simulink model "test_quadruped_troting"  (Simulink 9.2)
settings: Solver=VariableStepDiscrete  StartTime=0.0  StopTime=12  FixedStep=0.001  MaxStep=0.001  RelTol=1e-10  EnableMultiTasking=on
values from neighbouring files (symbols this model uses):
  Output_file_n = r_temp___(2)    [quadruped.m]
  Plant_inputs_num = r_temp___(1)    [quadruped.m]
  Plant_outputs_num = r_temp___(1)    [quadruped.m]
  RecurDyn_model_n = r_temp___(2)    [quadruped.m]
undefined symbols (not defined in the file): Matlab_version, Output_File, RecurDyn, RecurDyn_controltimestep, RecurDyn_model
(part 1 of 2)
settings Model: Creator=admin  LastModifiedBy=ahl19
settings OptimizationCC: ExpressionDepthLimit=2147483647
settings DebuggingCC: SolverPrmCheckMsg=warning
settings GRTTargetCC: CombineOutputUpdateFcns=on  GRTInterface=off

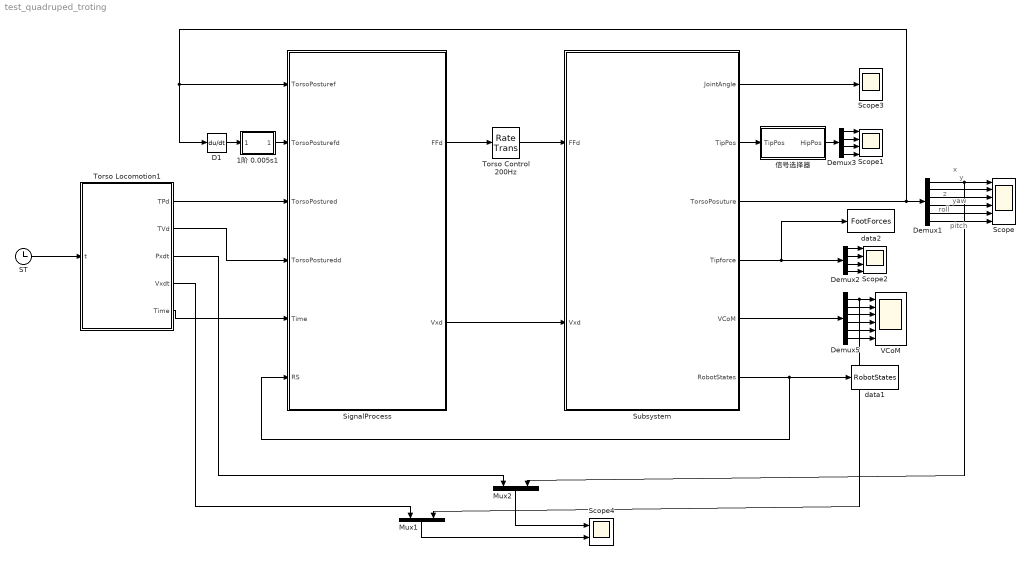
== system test_quadruped_troting ==
  note: x
  note: y
  note: z
  note: yaw
  note: roll
  note: pitch
  1阶 0.005s1 : Subsystem
  D1 : Derivative  CoefficientInTFapproximation=0.01
  Demux1 : Demux  Outputs=6
  Demux2 : Demux
  Demux3 : Demux
  Demux5 : Demux  Outputs=6
  Mux1 : Mux  Inputs=2
  Mux2 : Mux  Inputs=2
  ST : Clock
  Scope : Scope  NumInputPorts=6
  Scope1 : Scope  NumInputPorts=4
  Scope2 : Scope  NumInputPorts=4
  Scope3 : Scope
  Scope4 : Scope  NumInputPorts=2
  SignalProcess : MATLAB Function  TreatAsAtomicUnit=on
  Subsystem : Subsystem
  Torso Control 200Hz : RateTransition  OutPortSampleTime=0.005
  Torso Locomotion1 : MATLAB Function  TreatAsAtomicUnit=on
  VCoM : Scope  NumInputPorts=6
  data1 : ToWorkspace  VariableName=RobotStates  SaveFormat=Timeseries  SampleTime=-1
  data2 : ToWorkspace  VariableName=FootForces  SaveFormat=Timeseries  SampleTime=-1
  信号选择器 : MATLAB Function  TreatAsAtomicUnit=on
  wires:
  Subsystem/3(TorsoPosuture) -> Demux1/1, SignalProcess/1(TorsoPosturef), D1/1
  SignalProcess/1(FFd) -> Torso Control 200Hz/1
  Demux2/1 -> Scope2/1
  Demux2/2 -> Scope2/2
  Demux2/3 -> Scope2/3
  Demux2/4 -> Scope2/4
  Subsystem/4(Tipforce) -> Demux2/1, data2/1
  Subsystem/2(TipPos) -> 信号选择器/1(TipPos)
  Demux3/1 -> Scope1/1
  Demux3/2 -> Scope1/2
  Demux3/3 -> Scope1/3
  Demux3/4 -> Scope1/4
  Subsystem/1(JointAngle) -> Scope3/1
  信号选择器/1(HipPos) -> Demux3/1
  Torso Control 200Hz/1 -> Subsystem/1(FFd)
  Subsystem/6(RobotStates) -> data1/1, SignalProcess/6(RS)
  Subsystem/5(VCoM) -> Demux5/1
  Demux5/1 -> VCoM/1, Mux1/2
  Demux5/2 -> VCoM/2
  Demux5/3 -> VCoM/3
  Demux5/4 -> VCoM/4
  Demux5/5 -> VCoM/5
  Demux5/6 -> VCoM/6
  D1/1 -> 1阶 0.005s1/1(VT0)
  1阶 0.005s1/1(VT1) -> SignalProcess/2(TorsoPosturefd)
  SignalProcess/2(Vxd) -> Subsystem/2(Vxd)
  Demux1/1 -> Scope/1, Mux2/2
  Demux1/2 -> Scope/2
  Demux1/3 -> Scope/3
  Demux1/4 -> Scope/4
  Demux1/5 -> Scope/5
  Demux1/6 -> Scope/6
  Torso Locomotion1/5(Time) -> SignalProcess/5(Time)
  Torso Locomotion1/1(TPd) -> SignalProcess/3(TorsoPostured)
  Torso Locomotion1/2(TVd) -> SignalProcess/4(TorsoPosturedd)
  ST/1 -> Torso Locomotion1/1(t)
  Torso Locomotion1/3(Pxdt) -> Mux2/1
  Mux2/1 -> Scope4/1
  Torso Locomotion1/4(Vxdt) -> Mux1/1
  Mux1/1 -> Scope4/2

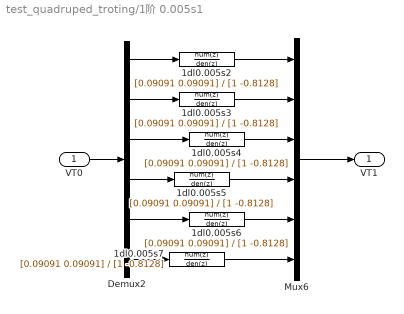
== system test_quadruped_troting/1阶 0.005s1 ==
  VT0 : Inport
  1dl0.005s{2..7} (6 alike) : DiscreteTransferFcn  Numerator=[0.09091 0.09091]  Denominator=[1 -0.8128]  SampleTime=0.001
  Demux2 : Demux  Outputs=6
  Mux6 : Mux  Inputs=6
  VT1 : Outport
  wires:
  Demux2/1 -> 1dl0.005s2/1
  Demux2/2 -> 1dl0.005s3/1
  Demux2/3 -> 1dl0.005s4/1
  Demux2/4 -> 1dl0.005s5/1
  Demux2/5 -> 1dl0.005s6/1
  Demux2/6 -> 1dl0.005s7/1
  1dl0.005s2/1 -> Mux6/1
  1dl0.005s4/1 -> Mux6/3
  1dl0.005s5/1 -> Mux6/4
  1dl0.005s6/1 -> Mux6/5
  1dl0.005s7/1 -> Mux6/6
  1dl0.005s3/1 -> Mux6/2
  Mux6/1 -> VT1/1
  VT0/1 -> Demux2/1

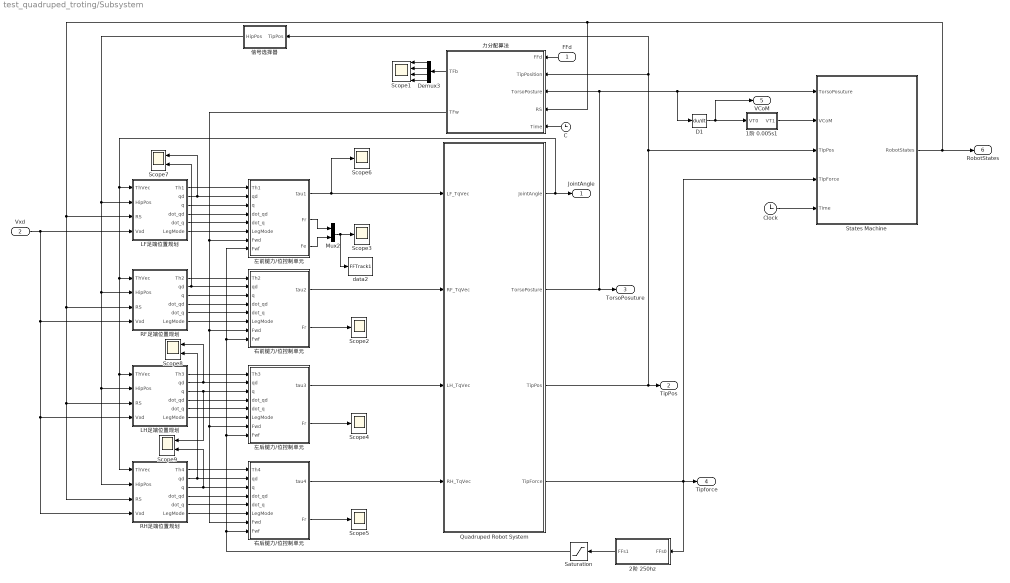
== system test_quadruped_troting/Subsystem ==
  FFd : Inport
  Vxd : Inport  Port=2
  1阶 0.005s1 : Subsystem
  2阶 250hz : Subsystem
  C : Clock
  Clock : Clock
  D1 : Derivative  CoefficientInTFapproximation=0.01
  Demux3 : Demux
  LF足端位置规划 : Subsystem
  LH足端位置规划 : Subsystem
  Mux2 : Mux  Inputs=2
  Quadruped Robot System : Subsystem
  RF足端位置规划 : Subsystem
  RH足端位置规划 : Subsystem
  Saturation : Saturate  UpperLimit=1500  LowerLimit=-1500
  Scope1 : Scope  NumInputPorts=4
  Scope{2..6} (5 alike) : Scope
  Scope7 : Scope  NumInputPorts=2
  Scope8 : Scope  NumInputPorts=2
  Scope9 : Scope  NumInputPorts=2
  States Machine : MATLAB Function  TreatAsAtomicUnit=on
  data2 : ToWorkspace  VariableName=FFTrack1  SaveFormat=Timeseries  SampleTime=-1
  信号选择器 : MATLAB Function  TreatAsAtomicUnit=on
  力分配算法 : MATLAB Function  TreatAsAtomicUnit=on
  右前腿力/位控制单元 : MATLAB Function  TreatAsAtomicUnit=on
  右后腿力/位控制单元 : MATLAB Function  TreatAsAtomicUnit=on
  左前腿力/位控制单元 : MATLAB Function  TreatAsAtomicUnit=on
  左后腿力/位控制单元 : MATLAB Function  TreatAsAtomicUnit=on
  JointAngle : Outport
  TipPos : Outport  Port=2
  TorsoPosuture : Outport  Port=3
  Tipforce : Outport  Port=4
  VCoM : Outport  Port=5
  RobotStates : Outport  Port=6
  wires:
  Quadruped Robot System/1(JointAngle) -> JointAngle/1, LF足端位置规划/1(ThVec), RF足端位置规划/1(ThVec), LH足端位置规划/1(ThVec), RH足端位置规划/1(ThVec)
  Quadruped Robot System/3(TipPos) -> TipPos/1, 信号选择器/1(TipPos), 力分配算法/2(TipPosition), States Machine/3(TipPos)
  Quadruped Robot System/2(TorsoPosture) -> TorsoPosuture/1, 力分配算法/3(TorsoPosture), States Machine/1(TorsoPosuture), D1/1
  Quadruped Robot System/4(TipForce) -> Tipforce/1, States Machine/4(TipForce), 2阶 250hz/1(FFs0)
  FFd/1 -> 力分配算法/1(FFd)
  C/1 -> 力分配算法/5(Time)
  左前腿力/位控制单元/1(tau1) -> Scope6/1, Quadruped Robot System/1(LF_TqVec)
  Demux3/1 -> Scope1/1
  Demux3/2 -> Scope1/2
  Demux3/3 -> Scope1/3
  Demux3/4 -> Scope1/4
  力分配算法/1(TFb) -> Demux3/1
  右前腿力/位控制单元/2(Fr) -> Scope2/1
  左后腿力/位控制单元/2(Fr) -> Scope4/1
  右后腿力/位控制单元/2(Fr) -> Scope5/1
  Mux2/1 -> Scope3/1, data2/1
  左前腿力/位控制单元/2(Fr) -> Mux2/1
  左前腿力/位控制单元/3(Fe) -> Mux2/2
  Clock/1 -> States Machine/5(Time)
  States Machine/1(RobotStates) -> RobotStates/1, LF足端位置规划/3(RS), LH足端位置规划/3(RS), RH足端位置规划/3(RS), RF足端位置规划/3(RS), 力分配算法/4(RS)
  LF足端位置规划/1(Th1) -> 左前腿力/位控制单元/1(Th1)
  LF足端位置规划/2(qd) -> Scope7/1, 左前腿力/位控制单元/2(qd)
  LF足端位置规划/3(q) -> 左前腿力/位控制单元/3(q)
  LF足端位置规划/4(dot_qd) -> 左前腿力/位控制单元/4(dot_qd)
  LF足端位置规划/5(dot_q) -> 左前腿力/位控制单元/5(dot_q)
  LF足端位置规划/6(LegMode) -> 左前腿力/位控制单元/6(LegMode)
  RF足端位置规划/1(Th2) -> 右前腿力/位控制单元/1(Th2)
  RF足端位置规划/2(qd) -> 右前腿力/位控制单元/2(qd), Scope7/2
  RF足端位置规划/3(q) -> 右前腿力/位控制单元/3(q)
  RF足端位置规划/4(dot_qd) -> 右前腿力/位控制单元/4(dot_qd)
  RF足端位置规划/5(dot_q) -> 右前腿力/位控制单元/5(dot_q)
  RF足端位置规划/6(LegMode) -> 右前腿力/位控制单元/6(LegMode)
  LH足端位置规划/1(Th3) -> 左后腿力/位控制单元/1(Th3)
  LH足端位置规划/2(qd) -> 左后腿力/位控制单元/2(qd), Scope8/1
  LH足端位置规划/3(q) -> 左后腿力/位控制单元/3(q), Scope9/1
  LH足端位置规划/4(dot_qd) -> 左后腿力/位控制单元/4(dot_qd)
  LH足端位置规划/5(dot_q) -> 左后腿力/位控制单元/5(dot_q)
  LH足端位置规划/6(LegMode) -> 左后腿力/位控制单元/6(LegMode)
  RH足端位置规划/1(Th4) -> 右后腿力/位控制单元/1(Th4)
  RH足端位置规划/2(qd) -> 右后腿力/位控制单元/2(qd), Scope8/2
  RH足端位置规划/3(q) -> 右后腿力/位控制单元/3(q), Scope9/2
  RH足端位置规划/4(dot_qd) -> 右后腿力/位控制单元/4(dot_qd)
  RH足端位置规划/5(dot_q) -> 右后腿力/位控制单元/5(dot_q)
  RH足端位置规划/6(LegMode) -> 右后腿力/位控制单元/6(LegMode)
  信号选择器/1(HipPos) -> LF足端位置规划/2(HipPos), RF足端位置规划/2(HipPos), LH足端位置规划/2(HipPos), RH足端位置规划/2(HipPos)
  力分配算法/2(TFw) -> 左前腿力/位控制单元/7(Fwd), 右前腿力/位控制单元/7(Fwd), 左后腿力/位控制单元/7(Fwd), 右后腿力/位控制单元/7(Fwd)
  Saturation/1 -> 右后腿力/位控制单元/8(Fwf), 左后腿力/位控制单元/8(Fwf), 右前腿力/位控制单元/8(Fwf), 左前腿力/位控制单元/8(Fwf)
  D1/1 -> 1阶 0.005s1/1(VT0), VCoM/1
  2阶 250hz/1(FFs1) -> Saturation/1
  1阶 0.005s1/1(VT1) -> States Machine/2(VCoM)
  Vxd/1 -> LF足端位置规划/4(Vxd), RF足端位置规划/4(Vxd), LH足端位置规划/4(Vxd), RH足端位置规划/4(Vxd)
  右前腿力/位控制单元/1(tau2) -> Quadruped Robot System/2(RF_TqVec)
  左后腿力/位控制单元/1(tau3) -> Quadruped Robot System/3(LH_TqVec)
  右后腿力/位控制单元/1(tau4) -> Quadruped Robot System/4(RH_TqVec)

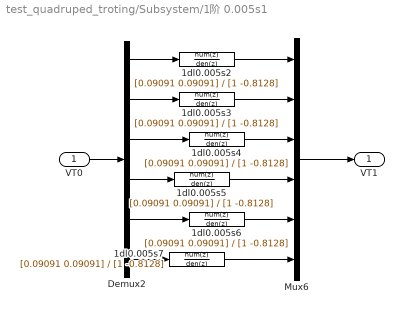
== system test_quadruped_troting/Subsystem/1阶 0.005s1 ==
  VT0 : Inport
  1dl0.005s{2..7} (6 alike) : DiscreteTransferFcn  Numerator=[0.09091 0.09091]  Denominator=[1 -0.8128]  SampleTime=0.001
  Demux2 : Demux  Outputs=6
  Mux6 : Mux  Inputs=6
  VT1 : Outport
  wires:
  Demux2/1 -> 1dl0.005s2/1
  Demux2/2 -> 1dl0.005s3/1
  Demux2/3 -> 1dl0.005s4/1
  Demux2/4 -> 1dl0.005s5/1
  Demux2/5 -> 1dl0.005s6/1
  Demux2/6 -> 1dl0.005s7/1
  1dl0.005s2/1 -> Mux6/1
  1dl0.005s4/1 -> Mux6/3
  1dl0.005s5/1 -> Mux6/4
  1dl0.005s6/1 -> Mux6/5
  1dl0.005s7/1 -> Mux6/6
  1dl0.005s3/1 -> Mux6/2
  Mux6/1 -> VT1/1
  VT0/1 -> Demux2/1

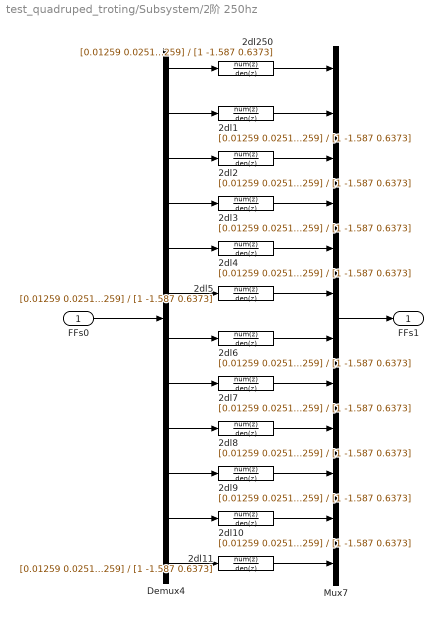
== system test_quadruped_troting/Subsystem/2阶 250hz ==
  FFs0 : Inport
  2dl{1..11,250} (12 alike) : DiscreteTransferFcn  Numerator=[0.01259 0.02519 0.01259]  Denominator=[1 -1.587 0.6373]  SampleTime=0.001
  Demux4 : Demux  Outputs=12
  Mux7 : Mux  Inputs=12
  FFs1 : Outport
  wires:
  FFs0/1 -> Demux4/1
  Mux7/1 -> FFs1/1
  Demux4/1 -> 2dl250/1
  Demux4/2 -> 2dl1/1
  Demux4/3 -> 2dl2/1
  Demux4/4 -> 2dl3/1
  Demux4/5 -> 2dl4/1
  Demux4/6 -> 2dl5/1
  Demux4/7 -> 2dl6/1
  Demux4/8 -> 2dl7/1
  Demux4/9 -> 2dl8/1
  Demux4/10 -> 2dl9/1
  Demux4/11 -> 2dl10/1
  Demux4/12 -> 2dl11/1
  2dl250/1 -> Mux7/1
  2dl1/1 -> Mux7/2
  2dl2/1 -> Mux7/3
  2dl3/1 -> Mux7/4
  2dl4/1 -> Mux7/5
  2dl5/1 -> Mux7/6
  2dl6/1 -> Mux7/7
  2dl7/1 -> Mux7/8
  2dl8/1 -> Mux7/9
  2dl9/1 -> Mux7/10
  2dl10/1 -> Mux7/11
  2dl11/1 -> Mux7/12

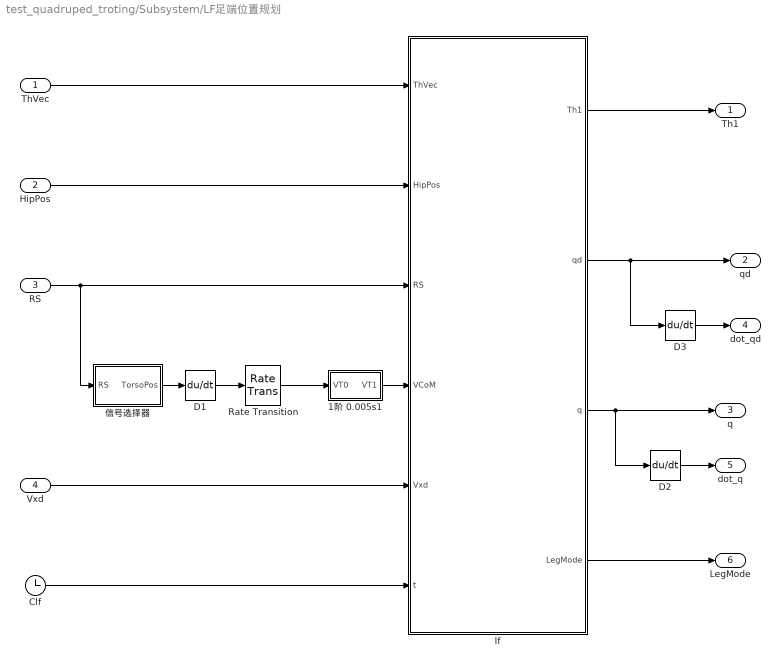
== system test_quadruped_troting/Subsystem/LF足端位置规划 ==
  ThVec : Inport
  HipPos : Inport  Port=2
  RS : Inport  Port=3
  Vxd : Inport  Port=4
  1阶 0.005s1 : Subsystem
  Clf : Clock
  D1 : Derivative  CoefficientInTFapproximation=0.01
  D2 : Derivative  CoefficientInTFapproximation=0.01
  D3 : Derivative  CoefficientInTFapproximation=0.01
  Rate Transition : RateTransition  OutPortSampleTime=0.002
  lf : MATLAB Function  TreatAsAtomicUnit=on
  信号选择器 : MATLAB Function  TreatAsAtomicUnit=on
  Th1 : Outport
  qd : Outport  Port=2
  q : Outport  Port=3
  dot_qd : Outport  Port=4
  dot_q : Outport  Port=5
  LegMode : Outport  Port=6
  wires:
  HipPos/1 -> lf/2(HipPos)
  ThVec/1 -> lf/1(ThVec)
  lf/1(Th1) -> Th1/1
  D2/1 -> dot_q/1
  D3/1 -> dot_qd/1
  Clf/1 -> lf/6(t)
  D1/1 -> Rate Transition/1
  lf/4(LegMode) -> LegMode/1
  RS/1 -> lf/3(RS), 信号选择器/1(RS)
  信号选择器/1(TorsoPos) -> D1/1
  lf/3(q) -> q/1, D2/1
  lf/2(qd) -> qd/1, D3/1
  Rate Transition/1 -> 1阶 0.005s1/1(VT0)
  1阶 0.005s1/1(VT1) -> lf/4(VCoM)
  Vxd/1 -> lf/5(Vxd)

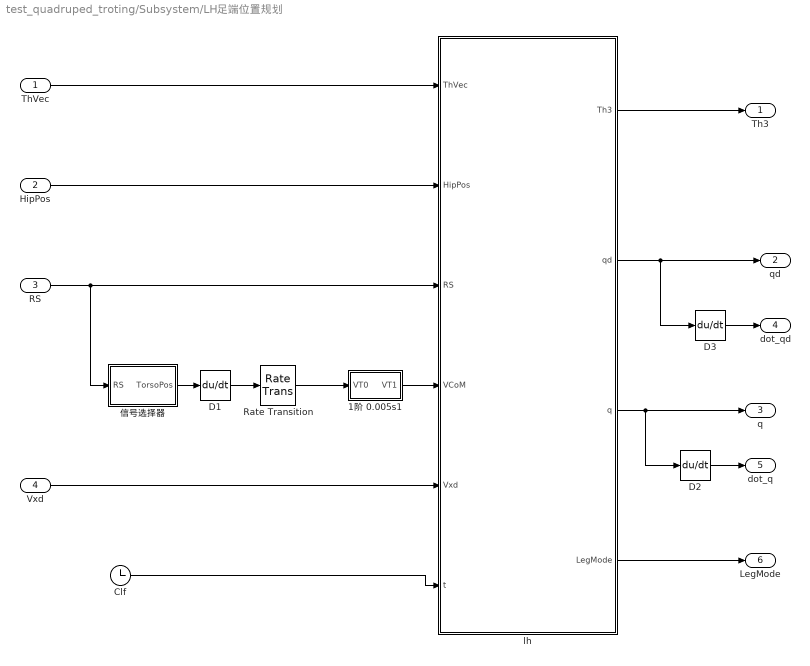
== system test_quadruped_troting/Subsystem/LH足端位置规划 ==
  ThVec : Inport
  HipPos : Inport  Port=2
  RS : Inport  Port=3
  Vxd : Inport  Port=4
  1阶 0.005s1 : Subsystem
  Clf : Clock
  D1 : Derivative  CoefficientInTFapproximation=0.01
  D2 : Derivative  CoefficientInTFapproximation=0.01
  D3 : Derivative  CoefficientInTFapproximation=0.01
  Rate Transition : RateTransition  OutPortSampleTime=0.002
  lh : MATLAB Function  TreatAsAtomicUnit=on
  信号选择器 : MATLAB Function  TreatAsAtomicUnit=on
  Th3 : Outport
  qd : Outport  Port=2
  q : Outport  Port=3
  dot_qd : Outport  Port=4
  dot_q : Outport  Port=5
  LegMode : Outport  Port=6
  wires:
  HipPos/1 -> lh/2(HipPos)
  ThVec/1 -> lh/1(ThVec)
  lh/1(Th3) -> Th3/1
  D2/1 -> dot_q/1
  D3/1 -> dot_qd/1
  Clf/1 -> lh/6(t)
  D1/1 -> Rate Transition/1
  lh/4(LegMode) -> LegMode/1
  RS/1 -> lh/3(RS), 信号选择器/1(RS)
  信号选择器/1(TorsoPos) -> D1/1
  lh/3(q) -> q/1, D2/1
  lh/2(qd) -> qd/1, D3/1
  Rate Transition/1 -> 1阶 0.005s1/1(VT0)
  1阶 0.005s1/1(VT1) -> lh/4(VCoM)
  Vxd/1 -> lh/5(Vxd)

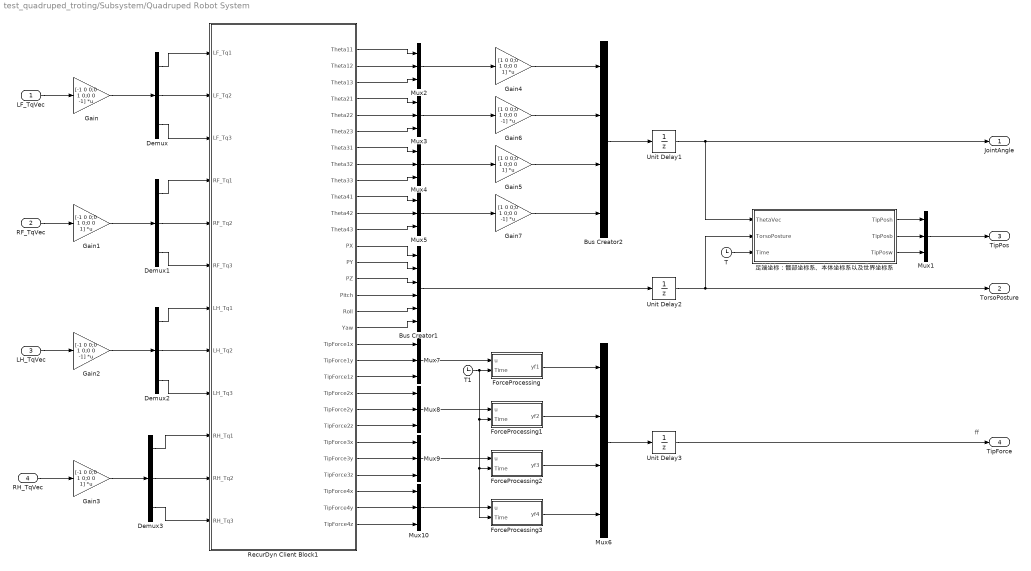
== system test_quadruped_troting/Subsystem/Quadruped Robot System ==
  note: ff
  LF_TqVec : Inport
  RF_TqVec : Inport  Port=2
  LH_TqVec : Inport  Port=3
  RH_TqVec : Inport  Port=4
  Bus Creator1 : BusCreator  Inputs=6
  Bus Creator2 : BusCreator  Inputs=4
  Demux{,1..3} (4 alike) : Demux  Outputs=3
  ForceProcessing : MATLAB Function  TreatAsAtomicUnit=on
  ForceProcessing1 : MATLAB Function  TreatAsAtomicUnit=on
  ForceProcessing2 : MATLAB Function  TreatAsAtomicUnit=on
  ForceProcessing3 : MATLAB Function  TreatAsAtomicUnit=on
  Gain : Gain  Gain=[-1 0 0;0 1 0;0 0 -1]  Multiplication=Matrix(K*u) (u vector)
  Gain1 : Gain  Gain=[-1 0 0;0 1 0;0 0 1]  Multiplication=Matrix(K*u) (u vector)
  Gain2 : Gain  Gain=[-1 0 0;0 1 0;0 0 -1]  Multiplication=Matrix(K*u) (u vector)
  Gain3 : Gain  Gain=[-1 0 0;0 1 0;0 0 1]  Multiplication=Matrix(K*u) (u vector)
  Gain4 : Gain  Gain=[1 0 0;0 1 0;0 0 1]  Multiplication=Matrix(K*u) (u vector)
  Gain5 : Gain  Gain=[1 0 0;0 1 0;0 0 1]  Multiplication=Matrix(K*u) (u vector)
  Gain6 : Gain  Gain=[1 0 0;0 1 0;0 0 -1]  Multiplication=Matrix(K*u) (u vector)
  Gain7 : Gain  Gain=[1 0 0;0 1 0;0 0 -1]  Multiplication=Matrix(K*u) (u vector)
  Mux{1..5,7..10} (9 alike) : Mux  Inputs=3
  Mux6 : Mux
  RecurDyn Client Block1 : Subsystem
      mask Display: image(imread('RecurDyn_IF3x_Client.jpg'))
  T : Clock
  T1 : Clock
  Unit Delay1 : UnitDelay  InitialCondition=[pi/2;pi/4;0;pi/2;pi/4;0;pi/2;pi/4;0;pi/2;pi/4;0]  SampleTime=0.001
  Unit Delay2 : UnitDelay  InitialCondition=[0;0.70;0;0;0;0]  SampleTime=0.001
  Unit Delay3 : UnitDelay  InitialCondition=[0;0;0;0;0;0;0;0;0;0;0;0]  SampleTime=0.001
  足端坐标：髋部坐标系、本体坐标系以及世界坐标系 : MATLAB Function  TreatAsAtomicUnit=on
  JointAngle : Outport
  TorsoPosture : Outport  Port=2
  TipPos : Outport  Port=3
  TipForce : Outport  Port=4
  wires:
  Bus Creator2/1 -> Unit Delay1/1
  Mux1/1 -> TipPos/1
  足端坐标：髋部坐标系、本体坐标系以及世界坐标系/1(TipPosh) -> Mux1/1
  足端坐标：髋部坐标系、本体坐标系以及世界坐标系/2(TipPosb) -> Mux1/2
  足端坐标：髋部坐标系、本体坐标系以及世界坐标系/3(TipPosw) -> Mux1/3
  Unit Delay1/1 -> JointAngle/1, 足端坐标：髋部坐标系、本体坐标系以及世界坐标系/1(ThetaVec)
  Unit Delay3/1 -> TipForce/1
  Unit Delay2/1 -> TorsoPosture/1, 足端坐标：髋部坐标系、本体坐标系以及世界坐标系/2(TorsoPosture)
  Mux7/1 -> ForceProcessing/1(u)
  Mux8/1 -> ForceProcessing1/1(u)
  Mux9/1 -> ForceProcessing2/1(u)
  Mux10/1 -> ForceProcessing3/1(u)
  Gain/1 -> Demux/1
  LF_TqVec/1 -> Gain/1
  RF_TqVec/1 -> Gain1/1
  LH_TqVec/1 -> Gain2/1
  RH_TqVec/1 -> Gain3/1
  Mux2/1 -> Gain4/1
  Bus Creator1/1 -> Unit Delay2/1
  Demux/2 -> RecurDyn Client Block1/2(LF_Tq2)
  RecurDyn Client Block1/1("Theta11   ") -> Mux2/1
  RecurDyn Client Block1/2("Theta12   ") -> Mux2/2
  RecurDyn Client Block1/3("Theta13   ") -> Mux2/3
  RecurDyn Client Block1/4("Theta21   ") -> Mux3/1
  RecurDyn Client Block1/5("Theta22   ") -> Mux3/2
  RecurDyn Client Block1/6("Theta23   ") -> Mux3/3
  Mux3/1 -> Gain6/1
  RecurDyn Client Block1/7("Theta31   ") -> Mux4/1
  RecurDyn Client Block1/8("Theta32   ") -> Mux4/2
  RecurDyn Client Block1/9("Theta33   ") -> Mux4/3
  RecurDyn Client Block1/10("Theta41   ") -> Mux5/1
  RecurDyn Client Block1/11("Theta42   ") -> Mux5/2
  RecurDyn Client Block1/12("Theta43   ") -> Mux5/3
  Mux4/1 -> Gain5/1
  Mux5/1 -> Gain7/1
  Demux1/2 -> RecurDyn Client Block1/5(RF_Tq2)
  Demux1/1 -> RecurDyn Client Block1/4(RF_Tq1)
  Demux1/3 -> RecurDyn Client Block1/6(RF_Tq3)
  Demux/1 -> RecurDyn Client Block1/1(LF_Tq1)
  Demux/3 -> RecurDyn Client Block1/3(LF_Tq3)
  Gain1/1 -> Demux1/1
  Demux2/2 -> RecurDyn Client Block1/8(LH_Tq2)
  Demux2/1 -> RecurDyn Client Block1/7(LH_Tq1)
  Demux2/3 -> RecurDyn Client Block1/9(LH_Tq3)
  Gain2/1 -> Demux2/1
  Demux3/2 -> RecurDyn Client Block1/11(RH_Tq2)
  Demux3/1 -> RecurDyn Client Block1/10(RH_Tq1)
  Demux3/3 -> RecurDyn Client Block1/12(RH_Tq3)
  Gain3/1 -> Demux3/1
  RecurDyn Client Block1/19(TipForce1x) -> Mux7/1
  RecurDyn Client Block1/20(TipForce1y) -> Mux7/2
  RecurDyn Client Block1/21(TipForce1z) -> Mux7/3
  RecurDyn Client Block1/22(TipForce2x) -> Mux8/1
  RecurDyn Client Block1/23(TipForce2y) -> Mux8/2
  RecurDyn Client Block1/24(TipForce2z) -> Mux8/3
  RecurDyn Client Block1/25(TipForce3x) -> Mux9/1
  RecurDyn Client Block1/26(TipForce3y) -> Mux9/2
  RecurDyn Client Block1/27(TipForce3z) -> Mux9/3
  RecurDyn Client Block1/28(TipForce4x) -> Mux10/1
  RecurDyn Client Block1/29(TipForce4y) -> Mux10/2
  RecurDyn Client Block1/30(TipForce4z) -> Mux10/3
  RecurDyn Client Block1/13("PX        ") -> Bus Creator1/1
  RecurDyn Client Block1/14("PY        ") -> Bus Creator1/2
  RecurDyn Client Block1/15("PZ        ") -> Bus Creator1/3
  RecurDyn Client Block1/16("Pitch     ") -> Bus Creator1/4
  RecurDyn Client Block1/17("Roll      ") -> Bus Creator1/5
  RecurDyn Client Block1/18("Yaw       ") -> Bus Creator1/6
  Gain4/1 -> Bus Creator2/1
  Gain6/1 -> Bus Creator2/2
  Gain5/1 -> Bus Creator2/3
  Gain7/1 -> Bus Creator2/4
  Mux6/1 -> Unit Delay3/1
  T/1 -> 足端坐标：髋部坐标系、本体坐标系以及世界坐标系/3(Time)
  ForceProcessing/1(yf1) -> Mux6/1
  ForceProcessing1/1(yf2) -> Mux6/2
  ForceProcessing2/1(yf3) -> Mux6/3
  ForceProcessing3/1(yf4) -> Mux6/4
  T1/1 -> ForceProcessing/2(Time), ForceProcessing1/2(Time), ForceProcessing2/2(Time), ForceProcessing3/2(Time)

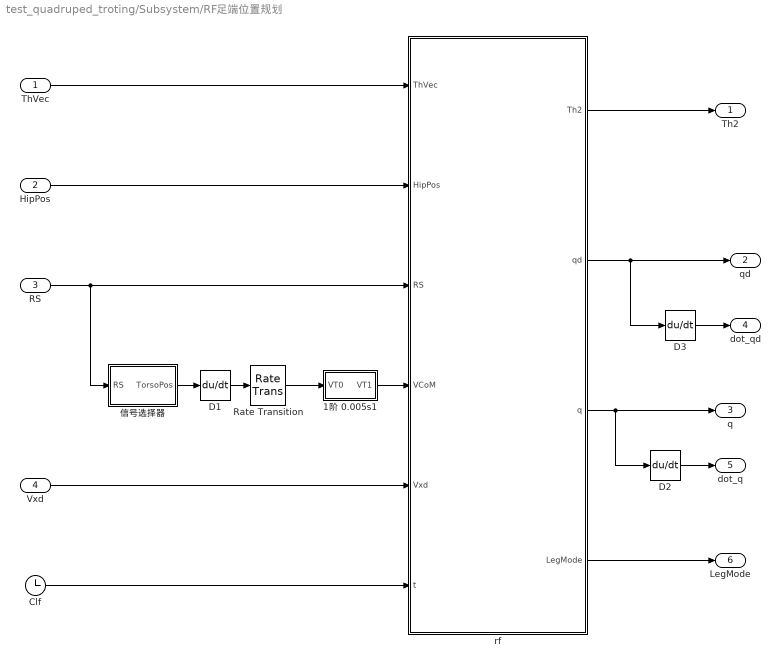
== system test_quadruped_troting/Subsystem/RF足端位置规划 ==
  ThVec : Inport
  HipPos : Inport  Port=2
  RS : Inport  Port=3
  Vxd : Inport  Port=4
  1阶 0.005s1 : Subsystem
  Clf : Clock
  D1 : Derivative  CoefficientInTFapproximation=0.01
  D2 : Derivative  CoefficientInTFapproximation=0.01
  D3 : Derivative  CoefficientInTFapproximation=0.01
  Rate Transition : RateTransition  OutPortSampleTime=0.002
  rf : MATLAB Function  TreatAsAtomicUnit=on
  信号选择器 : MATLAB Function  TreatAsAtomicUnit=on
  Th2 : Outport
  qd : Outport  Port=2
  q : Outport  Port=3
  dot_qd : Outport  Port=4
  dot_q : Outport  Port=5
  LegMode : Outport  Port=6
  wires:
  HipPos/1 -> rf/2(HipPos)
  ThVec/1 -> rf/1(ThVec)
  rf/1(Th2) -> Th2/1
  D2/1 -> dot_q/1
  D3/1 -> dot_qd/1
  Clf/1 -> rf/6(t)
  D1/1 -> Rate Transition/1
  rf/4(LegMode) -> LegMode/1
  RS/1 -> rf/3(RS), 信号选择器/1(RS)
  信号选择器/1(TorsoPos) -> D1/1
  rf/3(q) -> q/1, D2/1
  rf/2(qd) -> qd/1, D3/1
  Rate Transition/1 -> 1阶 0.005s1/1(VT0)
  1阶 0.005s1/1(VT1) -> rf/4(VCoM)
  Vxd/1 -> rf/5(Vxd)

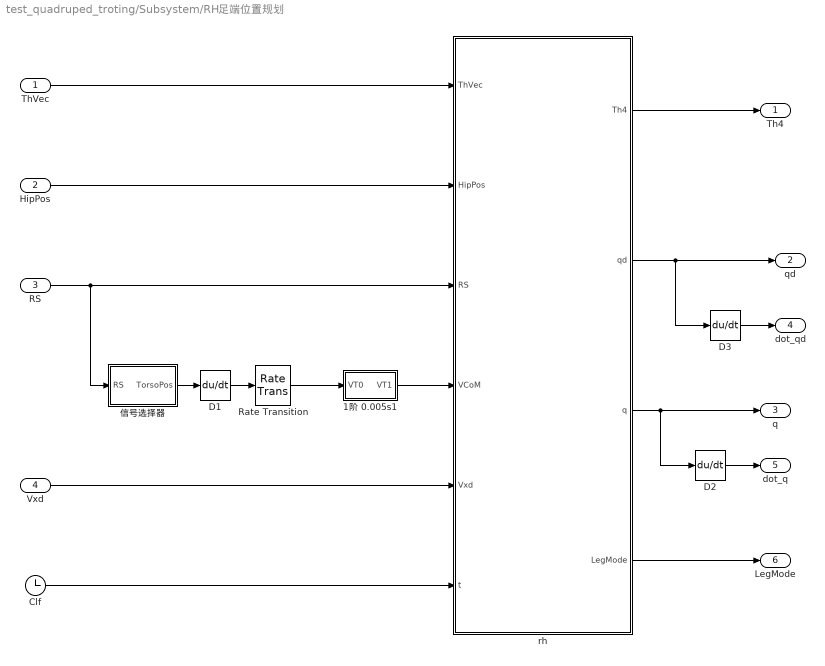
== system test_quadruped_troting/Subsystem/RH足端位置规划 ==
  ThVec : Inport
  HipPos : Inport  Port=2
  RS : Inport  Port=3
  Vxd : Inport  Port=4
  1阶 0.005s1 : Subsystem
  Clf : Clock
  D1 : Derivative  CoefficientInTFapproximation=0.01
  D2 : Derivative  CoefficientInTFapproximation=0.01
  D3 : Derivative  CoefficientInTFapproximation=0.01
  Rate Transition : RateTransition  OutPortSampleTime=0.002
  rh : MATLAB Function  TreatAsAtomicUnit=on
  信号选择器 : MATLAB Function  TreatAsAtomicUnit=on
  Th4 : Outport
  qd : Outport  Port=2
  q : Outport  Port=3
  dot_qd : Outport  Port=4
  dot_q : Outport  Port=5
  LegMode : Outport  Port=6
  wires:
  HipPos/1 -> rh/2(HipPos)
  ThVec/1 -> rh/1(ThVec)
  rh/1(Th4) -> Th4/1
  D2/1 -> dot_q/1
  D3/1 -> dot_qd/1
  Clf/1 -> rh/6(t)
  D1/1 -> Rate Transition/1
  rh/4(LegMode) -> LegMode/1
  RS/1 -> rh/3(RS), 信号选择器/1(RS)
  信号选择器/1(TorsoPos) -> D1/1
  rh/3(q) -> q/1, D2/1
  rh/2(qd) -> qd/1, D3/1
  Rate Transition/1 -> 1阶 0.005s1/1(VT0)
  1阶 0.005s1/1(VT1) -> rh/4(VCoM)
  Vxd/1 -> rh/5(Vxd)

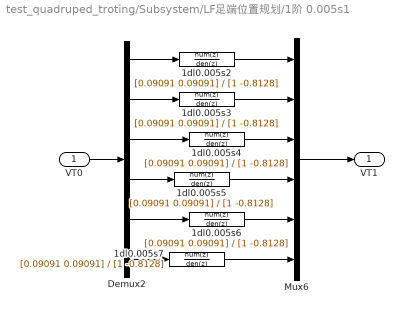
== system test_quadruped_troting/Subsystem/LF足端位置规划/1阶 0.005s1 ==
  VT0 : Inport
  1dl0.005s{2..7} (6 alike) : DiscreteTransferFcn  Numerator=[0.09091 0.09091]  Denominator=[1 -0.8128]  SampleTime=0.001
  Demux2 : Demux  Outputs=6
  Mux6 : Mux  Inputs=6
  VT1 : Outport
  wires:
  Demux2/1 -> 1dl0.005s2/1
  Demux2/2 -> 1dl0.005s3/1
  Demux2/3 -> 1dl0.005s4/1
  Demux2/4 -> 1dl0.005s5/1
  Demux2/5 -> 1dl0.005s6/1
  Demux2/6 -> 1dl0.005s7/1
  1dl0.005s2/1 -> Mux6/1
  1dl0.005s4/1 -> Mux6/3
  1dl0.005s5/1 -> Mux6/4
  1dl0.005s6/1 -> Mux6/5
  1dl0.005s7/1 -> Mux6/6
  1dl0.005s3/1 -> Mux6/2
  Mux6/1 -> VT1/1
  VT0/1 -> Demux2/1

== system test_quadruped_troting/Subsystem/LH足端位置规划/1阶 0.005s1 ==
  VT0 : Inport
  1dl0.005s{2..7} (6 alike) : DiscreteTransferFcn  Numerator=[0.09091 0.09091]  Denominator=[1 -0.8128]  SampleTime=0.001
  Demux2 : Demux  Outputs=6
  Mux6 : Mux  Inputs=6
  VT1 : Outport
  wires:
  Demux2/1 -> 1dl0.005s2/1
  Demux2/2 -> 1dl0.005s3/1
  Demux2/3 -> 1dl0.005s4/1
  Demux2/4 -> 1dl0.005s5/1
  Demux2/5 -> 1dl0.005s6/1
  Demux2/6 -> 1dl0.005s7/1
  1dl0.005s2/1 -> Mux6/1
  1dl0.005s4/1 -> Mux6/3
  1dl0.005s5/1 -> Mux6/4
  1dl0.005s6/1 -> Mux6/5
  1dl0.005s7/1 -> Mux6/6
  1dl0.005s3/1 -> Mux6/2
  Mux6/1 -> VT1/1
  VT0/1 -> Demux2/1

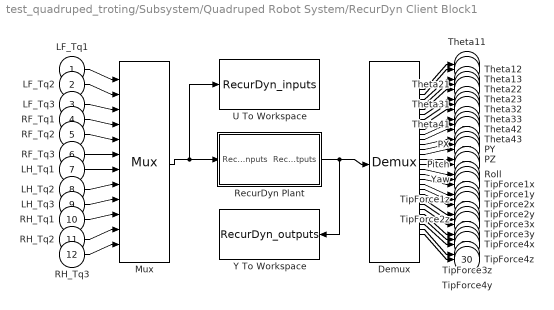
== system test_quadruped_troting/Subsystem/Quadruped Robot System/RecurDyn Client Block1 ==
  LF_Tq1 : Inport
  LF_Tq2 : Inport  Port=2
  LF_Tq3 : Inport  Port=3
  RF_Tq1 : Inport  Port=4
  RF_Tq2 : Inport  Port=5
  RF_Tq3 : Inport  Port=6
  LH_Tq1 : Inport  Port=7
  LH_Tq2 : Inport  Port=8
  LH_Tq3 : Inport  Port=9
  RH_Tq1 : Inport  Port=10
  RH_Tq2 : Inport  Port=11
  RH_Tq3 : Inport  Port=12
  Demux : Demux  Outputs=30
  Mux : Mux  Inputs=12
  RecurDyn Plant : Subsystem  mask(Recurdyn/Plant){RecurDyn_model_name=RecurDyn_model, Output_File_Name_=Output_File, RecurDyn_=RecurDyn, Matlab_version_=Matlab_version, RecurDyn_controltimestep_=RecurDyn_controltimestep, RecurDyn_step_=100, Waitingtime=1000, RecurDyn_static_=off, RecurDyn_show_=on, RecurDyn_ani_=on, Create_Output_Folder_=off}
      mask prompts: Output_File_Name_ "Output File Name"; RecurDyn_ "RecurDyn_install_directory"; Matlab_version_ "Matlab version"; RecurDyn_controltimestep_ "Sampling period"; RecurDyn_step_ "RecurDyn_step"; Waitingtime "Waiting time"; RecurDyn_static_ "Static analysis"; RecurDyn_show_ "RecurDyn_show"; RecurDyn_ani_ "RecurDyn_animation"; Create_Output_Folder_ "Create Output Folder"
      mask help:
      | Simulate any Recurdyn Dynamics Model in Recurdyn/Solver
      | Plant inputs and Plant outputs are transfered every sampling time
      | Here, sampling time is determined by sampling period (Control time step)
      mask Display: disp( 'Dynamic Model' )
  U To Workspace : ToWorkspace  VariableName=RecurDyn_inputs
  Y To Workspace : ToWorkspace  VariableName=RecurDyn_outputs
  "Theta11   " : Outport
  "Theta12   " : Outport  Port=2
  "Theta13   " : Outport  Port=3
  "Theta21   " : Outport  Port=4
  "Theta22   " : Outport  Port=5
  "Theta23   " : Outport  Port=6
  "Theta31   " : Outport  Port=7
  "Theta32   " : Outport  Port=8
  "Theta33   " : Outport  Port=9
  "Theta41   " : Outport  Port=10
  "Theta42   " : Outport  Port=11
  "Theta43   " : Outport  Port=12
  "PX        " : Outport  Port=13
  "PY        " : Outport  Port=14
  "PZ        " : Outport  Port=15
  "Pitch     " : Outport  Port=16
  "Roll      " : Outport  Port=17
  "Yaw       " : Outport  Port=18
  TipForce1x : Outport  Port=19
  TipForce1y : Outport  Port=20
  TipForce1z : Outport  Port=21
  TipForce2x : Outport  Port=22
  TipForce2y : Outport  Port=23
  TipForce2z : Outport  Port=24
  TipForce3x : Outport  Port=25
  TipForce3y : Outport  Port=26
  TipForce3z : Outport  Port=27
  TipForce4x : Outport  Port=28
  TipForce4y : Outport  Port=29
  TipForce4z : Outport  Port=30
  wires:
  RecurDyn Plant/1(RecurDyn_outputs) -> Demux/1, Y To Workspace/1
  Mux/1 -> RecurDyn Plant/1(" RecurDyn_inputs"), U To Workspace/1
  Demux/1 -> "Theta11   "/1
  Demux/2 -> "Theta12   "/1
  Demux/3 -> "Theta13   "/1
  Demux/4 -> "Theta21   "/1
  Demux/5 -> "Theta22   "/1
  Demux/6 -> "Theta23   "/1
  Demux/7 -> "Theta31   "/1
  Demux/8 -> "Theta32   "/1
  Demux/9 -> "Theta33   "/1
  Demux/10 -> "Theta41   "/1
  Demux/11 -> "Theta42   "/1
  Demux/12 -> "Theta43   "/1
  Demux/13 -> "PX        "/1
  Demux/14 -> "PY        "/1
  Demux/15 -> "PZ        "/1
  Demux/16 -> "Pitch     "/1
  Demux/17 -> "Roll      "/1
  Demux/18 -> "Yaw       "/1
  Demux/19 -> TipForce1x/1
  Demux/20 -> TipForce1y/1
  Demux/21 -> TipForce1z/1
  Demux/22 -> TipForce2x/1
  Demux/23 -> TipForce2y/1
  Demux/24 -> TipForce2z/1
  Demux/25 -> TipForce3x/1
  Demux/26 -> TipForce3y/1
  Demux/27 -> TipForce3z/1
  Demux/28 -> TipForce4x/1
  Demux/29 -> TipForce4y/1
  Demux/30 -> TipForce4z/1
  LF_Tq1/1 -> Mux/1
  LF_Tq2/1 -> Mux/2
  LF_Tq3/1 -> Mux/3
  RF_Tq1/1 -> Mux/4
  RF_Tq2/1 -> Mux/5
  RF_Tq3/1 -> Mux/6
  LH_Tq1/1 -> Mux/7
  LH_Tq2/1 -> Mux/8
  LH_Tq3/1 -> Mux/9
  RH_Tq1/1 -> Mux/10
  RH_Tq2/1 -> Mux/11
  RH_Tq3/1 -> Mux/12

== system test_quadruped_troting/Subsystem/RF足端位置规划/1阶 0.005s1 ==
  VT0 : Inport
  1dl0.005s{2..7} (6 alike) : DiscreteTransferFcn  Numerator=[0.09091 0.09091]  Denominator=[1 -0.8128]  SampleTime=0.001
  Demux2 : Demux  Outputs=6
  Mux6 : Mux  Inputs=6
  VT1 : Outport
  wires:
  Demux2/1 -> 1dl0.005s2/1
  Demux2/2 -> 1dl0.005s3/1
  Demux2/3 -> 1dl0.005s4/1
  Demux2/4 -> 1dl0.005s5/1
  Demux2/5 -> 1dl0.005s6/1
  Demux2/6 -> 1dl0.005s7/1
  1dl0.005s2/1 -> Mux6/1
  1dl0.005s4/1 -> Mux6/3
  1dl0.005s5/1 -> Mux6/4
  1dl0.005s6/1 -> Mux6/5
  1dl0.005s7/1 -> Mux6/6
  1dl0.005s3/1 -> Mux6/2
  Mux6/1 -> VT1/1
  VT0/1 -> Demux2/1

== system test_quadruped_troting/Subsystem/RH足端位置规划/1阶 0.005s1 ==
  VT0 : Inport
  1dl0.005s{2..7} (6 alike) : DiscreteTransferFcn  Numerator=[0.09091 0.09091]  Denominator=[1 -0.8128]  SampleTime=0.001
  Demux2 : Demux  Outputs=6
  Mux6 : Mux  Inputs=6
  VT1 : Outport
  wires:
  Demux2/1 -> 1dl0.005s2/1
  Demux2/2 -> 1dl0.005s3/1
  Demux2/3 -> 1dl0.005s4/1
  Demux2/4 -> 1dl0.005s5/1
  Demux2/5 -> 1dl0.005s6/1
  Demux2/6 -> 1dl0.005s7/1
  1dl0.005s2/1 -> Mux6/1
  1dl0.005s4/1 -> Mux6/3
  1dl0.005s5/1 -> Mux6/4
  1dl0.005s6/1 -> Mux6/5
  1dl0.005s7/1 -> Mux6/6
  1dl0.005s3/1 -> Mux6/2
  Mux6/1 -> VT1/1
  VT0/1 -> Demux2/1

== system test_quadruped_troting/Subsystem/Quadruped Robot System/RecurDyn Client Block1/RecurDyn Plant ==
  " RecurDyn_inputs" : Inport
  S-Function : S-Function  FunctionName=recurdyn_client_9_1  Parameters=RecurDyn_controltimestep_,RecurDyn_model_name,RecurDyn_,RecurDyn_static_,RecurDyn_step_,RecurDyn_show_,RecurDyn_ani_,Matlab_version_,RecurDyn_model_n,Plant_inputs_num,Plant_outputs_num,Waitingtime,Create_Output_Folder_,Output_File_Name_,Output_file_n  SFunctionDeploymentMode=off  EnableBusSupport=off
  RecurDyn_outputs : Outport  InitialOutput=0
  wires:
  S-Function/1 -> RecurDyn_outputs/1
  " RecurDyn_inputs"/1 -> S-Function/1

== matlab function Subsystem/Quadruped Robot System/ForceProcessing1 ==
  data: u input double; yf2 output double; Time input double
function yf2 = fp(u, Time)
% 处理足端力，y方向只提供大等于零的力
if Time<=0.001
    yf2 = zeros(3,1);
else
    yf2 = [1 0 0;0 (u(2)>=0) 0;0 0 1]*u;
end

end

== matlab function Subsystem/Quadruped Robot System/ForceProcessing ==
  data: u input double; yf1 output double; Time input double
function yf1 = fp(u, Time)
% 处理足端力，y方向只提供大等于零的力
if Time<=0.001
    yf1 = zeros(3,1);
else
    yf1 = [1 0 0;0 (u(2)>=0) 0;0 0 1]*u;
end

end

== matlab function Subsystem/Quadruped Robot System/ForceProcessing2 ==
  data: u input double; yf3 output double; Time input double
function yf3 = fp(u, Time)
% 处理足端力，y方向只提供大等于零的力
if Time<=0.001
    yf3 = zeros(3,1);
else
    yf3 = [1 0 0;0 (u(2)>=0) 0;0 0 1]*u;
end

end

== matlab function Subsystem/Quadruped Robot System/ForceProcessing3 ==
  data: u input double; yf4 output double; Time input double
function yf4 = fp(u, Time)
% 处理足端力，y方向只提供大等于零的力
if Time<=0.001
    yf4 = zeros(3,1);
else
    yf4 = [1 0 0;0 (u(2)>=0) 0;0 0 1]*u;
end

end

== matlab function Subsystem/力分配算法 ==
  data: FFd input double; TipPosition input double; TorsoPosture input double; RS input double; Time input double; TFb output double; TFw output double
function [TFb, TFw] = fdA(FFd,  TipPosition, TorsoPosture,  RS, Time)

%% 力分配算法：在惯性坐标系下进行
% FFD：本体在操作空间受到的等效控制力旋量，由规划层确定
% TipPosition：足端在髋部固连坐标系，本体固连坐标系以及原点在本体质心处的惯性系下的位置
% TorsoPosture：本体在惯性系下的绝对位置和姿态
% mode：四足支撑或两足之城
% time：仿真时间

% BY ZPP
% 20171124

%% 设置仿真输入初始值
if Time<=0.001
    TorsoPosture = [0; 0.70; 0; 0;0;0];
end

%% 模型参数
% 重力加速度
g = 9.80665;
% 本体质量
Mb = 50;
Mleg = 1.0+1.5+0.5;

%本体尺寸的一半
L = 0.425; W = 0.19; H = -0.10;
% 髋部安装点在本体固连坐标系中的坐标
A1 = [L -H -W]';
A2 = [L -H W]';
A3 = [-L -H -W]';
A4 = [-L -H W]';
AA = [A1;A2;A3;A4];

%% 本体姿态角：Y-pitch / X-roll / Z-yaw
alpha = TorsoPosture(6); beta = TorsoPosture(4); gama = TorsoPosture(5);
R0 = [cos(alpha)*cos(beta)  cos(alpha)*sin(beta)*sin(gama)-sin(alpha)*cos(gama)  cos(alpha)*sin(beta)*cos(gama)+sin(alpha)*sin(gama);...
         sin(alpha)*cos(beta)  sin(alpha)*sin(beta)*sin(gama)+cos(alpha)*cos(gama)  sin(alpha)*sin(beta)*cos(gama)-cos(alpha)*sin(gama);...
         -sin(beta)  cos(beta)*sin(gama)  cos(beta)*cos(gama)];
R1234 = blkdiag(R0,R0,R0,R0);

%% 力分配所需参数
% Fxd = 0;
% Fyd = 0 + (Mb+4*Mleg)*g;
% Fzd = 0;
% Txd = 0;
% Tyd = 0;
% Tzd = 0;
Fxd = FFd(1);
Fyd = FFd(2) + (Mb+4*Mleg)*g;
Fzd = FFd(3);

Txd = FFd(5);
Tyd = FFd(4);
Tzd = FFd(6);


% TipPosw1 = TipPosition(25:27);
X1 = TipPosition(25);
Y1 = TipPosition(26);
Z1 = TipPosition(27);
% TipPosw2 = TipPosition(28:30);
X2 = TipPosition(28);
Y2 = TipPosition(29);
Z2 = TipPosition(30);
% TipPosw3 = TipPosition(31:33);
X3 = TipPosition(31);
Y3 = TipPosition(32);
Z3 = TipPosition(33);
% TipPosw4 = TipPosition(34:36);
X4 = TipPosition(34);
Y4 = TipPosition(35);
Z4 = TipPosition(36);

% TipPosh0 = [0;-0.70;-0.09; 0;-0.70;+0.09; 0;-0.70;-0.09; 0;-0.70;+0.09];
% TipPosw0 = R1234*(TipPosh0+AA);
% 
% X1 = TipPosw0(1);
% Y1 = TipPosw0(2);
% Z1 = TipPosw0(3);
% 
% X2 = TipPosw0(4);
% Y2 = TipPosw0(5);
% Z2 = TipPosw0(6);
% 
% X3 = TipPosw0(7);
% Y3 = TipPosw0(8);
% Z3 = TipPosw0(9);
% 
% X4 = TipPosw0(10);
% Y4 = TipPosw0(11);
% Z4 = TipPosw0(12);


%% 选择支撑模式
y = RS(20);
if y==1  % 1/4腿支撑
    N = 1;
else  % y==0 ： 2/3腿支撑
    N = 2;
end

% %% 选择支撑模式
% if RS==14  % 1/4腿支撑
%     N = 1;
% elseif RS==23  % 2/3腿支撑
%     N = 2;
% elseif RS==1234  % 四足支撑
%     N = 3;
% else   % 其他情况
%     N=4;
% end
% N=3;

% dt = mod(Time,0.6);
% if dt>=0 && dt<0.3
%     N = 1;
% else
%     N = 2;
% end

%%  不同支撑模式下的力分配算法
switch N
    case 1
%%%%%%%%%%%%%%%%%%%%%%%%%%%%%%%%%%%%%%%%%%%%%%%%%%%%%%%%%%%%%%%%%%%%%%%%%%%%%%        
        FFFd = [Fxd;  Fyd;  (Txd-Mleg*g*(Z1+Z2+Z3+Z4));  Tyd;  (Tzd++Mleg*g*(X1+X2+X3+X4));  0];
        % 添加约束：内力为零
        A = [          eye(2)   [0 0]'                     eye(2)    [0 0]';...
               [0 -Z1 Y1;Z1 0 -X1;-Y1 X1 0]     [0 -Z4 Y4;Z4 0 -X4;-Y4 X4 0];...
               [(X1-X4)  (Y1-Y4)  (Z1-Z4)  -(X1-X4)  -(Y1-Y4)  -(Z1-Z4)]         ];

        rkA = rank(A);
        if (rkA<6)
            temp14 = [Fxd/2; Fyd/2; 0; Fxd/2; Fyd/2; 0];
        else
            temp14 = A\FFFd;
        end
        
        TFw=[temp14(1);temp14(2);temp14(3);0;0;0;0;0;0;temp14(4);temp14(5);temp14(6)];
        TFb = (R1234')*TFw;
%             the=abs(atan((Z1-Z4)/(X1-X4)));
%             A=[cos(the),0,-sin(the),cos(the),0,-sin(the)
%                  0,1,0,0,1,0
%                  Y1*sin(the),-Z1*cos(the)-X1*sin(the),Y1*cos(the),Y4*sin(the),-Z4*cos(the)-X4*sin(the),Y4*cos(the)
%                  Z1,0,-X1,Z4,0,-X4
%                  -Y1*cos(the),X1*cos(the)-Z1*sin(the),Y1*sin(the),-Y4*cos(the),X4*cos(the)-Z4*sin(the),Y4*sin(the) 
%                  X4-X1,Y4-Y1,Z4-Z1,X1-X4,Y1-Y4,Z1-Z4];
%              
%              temp14=A\[Fxd*cos(the)-Fzd*sin(the);   Fyd;   Txd*cos(the)-Tzd*sin(the)-Mleg*g*((Z1+Z2+Z3+Z4)*cos(the)+(X1+X2+X3+X4)*sin(the));   Tyd;   Txd*sin(the)+Tzd*cos(the)+Mleg*g*((X1+X2+X3+X4)*cos(the)-(Z1+Z2+Z3+Z4)*sin(the));   0];
%              TFw=[temp14(1);temp14(2);temp14(3);0;0;0;0;0;0;temp14(4);temp14(5);temp14(6)];
%              TFb = (R1234')*TFw;
        
    case 2
%%%%%%%%%%%%%%%%%%%%%%%%%%%%%%%%%%%%%%%%%%%%%%%%%%%%%%%%%%%%%%%%%%%%%%%%%%%%%%
        FFFd = [Fxd;  Fyd;  (Txd-Mleg*g*(Z1+Z2+Z3+Z4));  Tyd;  (Tzd++Mleg*g*(X1+X2+X3+X4));  0];
        % 添加约束：内力为零
        A = [          eye(2)   [0 0]'                     eye(2)    [0 0]';...
               [0 -Z2 Y2;Z2 0 -X2;-Y2 X2 0]     [0 -Z3 Y3;Z3 0 -X3;-Y3 X3 0];...
               [(X2-X3)  (Y2-Y3)  (Z2-Z3)  -(X2-X3)  -(Y2-Y3)  -(Z2-Z3)]          ];
        
        rkA = rank(A);
        if (rkA<6)
            temp23 = [Fxd/2; Fyd/2; 0; Fxd/2; Fyd/2; 0];
        else
            temp23 = A\FFFd;
        end
   
        TFw=[0;0;0;temp23(1);temp23(2);temp23(3);temp23(4);temp23(5);temp23(6);0;0;0];                                  
        TFb = (R1234')*TFw;

%             the=abs(atan((Z2-Z3)/(X2-X3)));
%             A=[cos(the),0,sin(the),cos(the),0,sin(the)
%                  0,1,0,0,1,0
%                  -Y2*sin(the),-Z2*cos(the)+X2*sin(the),Y2*cos(the),-Y3*sin(the),-Z3*cos(the)+X3*sin(the),Y3*cos(the)
%                  Z2,0,-X2,Z3,0,-X3
%                 -Y2*cos(the),X2*cos(the)+Z2*sin(the),-Y2*sin(the),-Y3*cos(the),X3*cos(the)+Z3*sin(the),-Y3*sin(the) 
%                 X3-X2,Y3-Y2,Z3-Z2,X2-X3,Y2-Y3,Z2-Z3];
%             
%             temp23=A\[Fxd*cos(the)+Fzd*sin(the);   Fyd;   Txd*cos(the)+Tzd*sin(the)-Mleg*g*((Z1+Z2+Z3+Z4)*cos(the)-(X1+X2+X3+X4)*sin(the));   Tyd;   -Txd*sin(the)+Tzd*cos(the)+Mleg*g*((X1+X2+X3+X4)*cos(the)+(Z1+Z2+Z3+Z4)*sin(the));   0];
%             TFw=[0;0;0;temp23(1);temp23(2);temp23(3);temp23(4);temp23(5);temp23(6);0;0;0];
%             TFb = (R1234')*TFw;
         
    case 3
%%%%%%%%%%%%%%%%%%%%%%%%%%%%%%%%%%%%%%%%%%%%%%%%%%%%%%%%%%%%%%%%%%%%%%%%%%%%%%
        FFFd = [Fyd;   Txd-Mleg*g*(Z1+Z2+Z3+Z4);   Tzd+Mleg*g*(X1+X2+X3+X4);   Mleg*g*(X1-X2+X3-X4-Z1-Z2+Z3+Z4);   Fxd;   0;   0;   Tyd;   Fzd;   0;0;0];
        A=[ 1,       1,       1,       1,       0,       0,       0,        0,       0,       0,       0,       0;
              -Z1,     -Z2,     -Z3,     -Z4,       0,       0,       0,       0,      Y1,      Y2,      Y3,      Y4;
              X1,      X2,      X3,      X4,     -Y1,     -Y2,     -Y3,     -Y4,       0,       0,       0,       0;
              X1 - Z1, - X2 - Z2, X3 + Z3, Z4 - X4,     -Y1,      Y2,     -Y3,      Y4,      Y1,      Y2,     -Y3,     -Y4;
               0,       0,       0,       0,       1,       1,       1,       1,       0,       0,       0,       0;
              Y3 - Y1,       0, Y1 - Y3,       0, X3 - X1,       0, X1 - X3,       0, Z3 - Z1,       0, Z1 - Z3,       0;
             0, Y4 - Y2,       0, Y2 - Y4,       0, X4 - X2,       0, X2 - X4,       0, Z4 - Z2,       0, Z2 - Z4;
             0,       0,       0,       0,      Z1,      Z2,      Z3,      Z4,     -X1,     -X2,     -X3,     -X4;
             0,       0,       0,       0,       0,       0,       0,       0,       1,       1,       1,       1;
             Y2 - Y1, Y1 - Y2,       0,       0, X2 - X1, X1 - X2,       0,       0, Z2 - Z1, Z1 - Z2,       0,       0;
            0,       0, Y4 - Y3, Y3 - Y4,       0,       0, X4 - X3, X3 - X4,       0,       0, Z4 - Z3, Z3 - Z4;  
            0, Y3 - Y2, Y2 - Y3,       0,       0, X3 - X2, X2 - X3,       0,       0, Z3 - Z2, Z2 - Z3,       0];
                
        temp1234 = A\FFFd;
        TFw = [temp1234(5);temp1234(1);temp1234(9);  temp1234(6);temp1234(2);temp1234(10);  temp1234(7);temp1234(3);temp1234(11);  temp1234(8);temp1234(4);temp1234(12)];
        TFb = (R1234')*TFw;
        
    otherwise
        TFw = zeros(12,1);
        TFb = zeros(12,1);
        
%%%%%%%%%%%%%%%%%%%%%%%%%%%%%%%%%%%%%%%%%%%%%%%%%%%%%%%%%%%%%%%%%%%%%%%%%%%%%          
end

%% 考虑摩擦锥约束
% uu = 0.80;


end

== matlab function Subsystem/Quadruped Robot System/足端坐标：髋部坐标系、本体坐标系以及世界坐标系 ==
  data: ThetaVec input double; TipPosh output double; TipPosb output double; TorsoPosture input double; TipPosw output double; Time input double
function [TipPosh,TipPosb, TipPosw] = fk(ThetaVec, TorsoPosture, Time)

%% Notes
% 惯性系或世界坐标系：以机器人前进方向为【+X】，竖直向上为【+Y】，【+Z】由右手法则确定
% 本体固连坐标系：原点在质心处或几何中心，初始方向与惯性系一致
% 在髋部安装点处建立固连坐标系（方向与本体固连坐标系一致），计算足端位置（以下的顺序均为：左前、右前、左后、右后）

% BY ZPP
% 20171122

%% 设置仿真初值
if Time<=0.001
    ThetaVec = [pi/2;pi/4;0; pi/2;pi/4;0; pi/2;pi/4;0; pi/2;pi/4;0];
    TorsoPosture = [0; 0.70; 0;0;0;0];
end

%% 设置模型参数

% 重力加速度
g = 9.80665;

%本体尺寸的一半
L = 0.425; W = 0.19; H = -0.10 ;
% 本体质量
Mb = 50;

% 髋部安装点在本体固连坐标系中的坐标
A1 = [L -H -W]';
A2 = [L -H W]';
A3 = [-L -H -W]';
A4 = [-L -H W]';

Ab= [A1;A2;A3;A4];

% 单腿各连杆长度和质量
L1 = 0.35*sqrt(2);      % M1 = 1.0;
L2 = 0.35*sqrt(2);      % M2 = 1.5;
R3 = 0.06;                  % M3 = 0.5;

%% 输入关节角度
th11 = ThetaVec(1);
th12 = ThetaVec(2);
th13 = ThetaVec(3);

th21 = ThetaVec(4);
th22 = ThetaVec(5);
th23 = ThetaVec(6);

th31 = ThetaVec(7);
th32 = ThetaVec(8);
th33 = ThetaVec(9);

th41 = ThetaVec(10);
th42 = ThetaVec(11);
th43 = ThetaVec(12);

%% 正运动学1：计算髋部固连坐标系下足端的位置
x1 = L1*cos(th11 - th12) - L2*cos(th12);
y1 = - cos(th13)*(L2*sin(th12) + L1*sin(th11 - th12));
z1 = - sin(th13)*(L2*sin(th12) + L1*sin(th11 - th12));

x2 = L1*cos(th21 - th22) - L2*cos(th22);
y2 = - cos(th23)*(L2*sin(th22) + L1*sin(th21 - th22));
z2 = sin(th23)*(L2*sin(th22) + L1*sin(th21 - th22));

x3 = L1*cos(th31 - th32) - L2*cos(th32);
y3 = - cos(th33)*(L2*sin(th32) + L1*sin(th31 - th32));
z3 = - sin(th33)*(L2*sin(th32) + L1*sin(th31 - th32));

x4 = L1*cos(th41 - th42) - L2*cos(th42);
y4 = - cos(th43)*(L2*sin(th42) + L1*sin(th41 - th42));
z4 = sin(th43)*(L2*sin(th42) + L1*sin(th41 - th42));

TipPosh = [x1 y1 z1 x2 y2 z2 x3 y3 z3 x4 y4 z4]';

%% 正运动学2：计算本体固连坐标系下足端的位置
TipPosb = TipPosh + Ab;

%% 正运动学3：计算原点在本体质心处的惯性系下足端的位置
% 本体姿态角：Y-pitch / X-roll / Z-yaw
alpha = TorsoPosture(6); beta = TorsoPosture(4); gama = TorsoPosture(5);
RR = [cos(alpha)*cos(beta)  cos(alpha)*sin(beta)*sin(gama)-sin(alpha)*cos(gama)  cos(alpha)*sin(beta)*cos(gama)+sin(alpha)*sin(gama);...
         sin(alpha)*cos(beta)  sin(alpha)*sin(beta)*sin(gama)+cos(alpha)*cos(gama)  sin(alpha)*sin(beta)*cos(gama)-cos(alpha)*sin(gama);...
         -sin(beta)  cos(beta)*sin(gama)  cos(beta)*cos(gama)];
Rmat = blkdiag(RR,RR,RR,RR);
TipPosw = Rmat*TipPosb;

end

== matlab function SignalProcess ==
  data: TorsoPosturef input double; TorsoPosturefd input double; TorsoPostured input double; FFd output double; TorsoPosturedd input double; Time input double; RS input double; Vxd output double
function [ FFd, Vxd] = fcn(TorsoPosturef, TorsoPosturefd, TorsoPostured, TorsoPosturedd, Time, RS)
% 计算本体在操作空间受到的等效力/力矩

%% 反馈信息
if Time<=0.001
    TorsoPosturef = [0; 0.70; 0;0;0;0];
    TorsoPosturefd = zeros(6,1);
end

% 调整期望姿态与仿真中姿态角的顺序：XYZ  >> YXZ
Rxyz = eye(3); Rryp = [0 1 0;1 0 0;0 0 1];
TorsoPostured =  (blkdiag(Rxyz,Rryp))*TorsoPostured;
TorsoPosturedd =  (blkdiag(Rxyz,Rryp))*TorsoPosturedd;
% 本体前向速度规划
Vxd = TorsoPosturedd(1);

%% PD参数设置
kpx = 3500;    kdx = 1000;

kpy = 500;      kdy = 100;  % 无实际意义
kpz = 200;    kdz = 100;  % 无实际意义


% 真实的顺序        
kppitch = 3000;          % Yaw （Y）
kproll = 3500;             % Roll（X）
kpyaw = 3000;            % Pitch（Z）

kdpitch = 500;           
kdroll = 1000;                
kdyaw = 500;              

Kp = diag([kpx,kpy,kpz,kppitch,kproll,kpyaw]);
Kd = diag([kdx,kdy,kdz,kdpitch,kdroll,kdyaw]);

%% 计算控制量（具有力的量纲）
FFd = diag([1 1 1 1 1 1])*Kp*(TorsoPostured-TorsoPosturef) + Kd*(TorsoPosturedd-TorsoPosturefd);

%% 基于本体高度以及速度的弹跳切换控制

% 本体高度及速度状态信息
PYf = TorsoPosturef(2);
VYf = TorsoPosturefd(2);

% 设置期望的起跳高度以及起跳速度
% Hlod = 0.65; % 对应腿长为0.75m
Vlod = 0.40;

% 支撑腿状态信息
% Swg2Sup1 = RS(7);
NumTDL = RS(19);
NumAccSwitch = RS(35);
% VYf = temp;
if (NumTDL<=2) && (NumTDL>=1) 
    % 至少有一足支撑且未达到起跳高度，则规划Y方向上的期望足端力
    if (NumAccSwitch >=1) || (VYf > Vlod)
        accd = - 0.5;
    else
        accd = 12;
    end
else
    accd = - 0.5;
end

FFyd = 50*accd; % 期望加速度 Mb*accd
% FFyd = 300;
FFd = [FFd(1); FFyd; FFd(3:6)];



end

== matlab function Subsystem/信号选择器 ==
  data: TipPos input double; HipPos output double
function HipPos  = SS(TipPos)

%% 
HipPos = TipPos(1:12);


end

== matlab function Torso Locomotion1 ==
  data: TPd output double; t input double; TVd output double; Pxdt output double; Vxdt output double; Time output double
function [TPd, TVd, Pxdt, Vxdt, Time]  = Planning(t)
% 主要规划四足机器人本体前向速度

%% 设置相关参数
% 最大前向速度为【1m/s】
vxd = 1.0;
t0 = 3;       % 之前原地
t1 = 8;     % 之前加速，加速时间（t1-t0）
t2 = 15;    % 之前匀速
t3 = 55;    % 之前减速，减速时间（t3-t2）
t4 = 65;    % 之前原地
t5 = 45;    % 之前反向加速，反向加速时间（t5-t4）
t6 = 50;    % 之前反向匀速
t7= 60;     % 之前反向减速，反向减速时间（t7-t6），之后原地

a0 = (t0^2*vxd*(t0 - 3*t1))/((t0 - t1)*(t0^2 - 2*t0*t1 + t1^2));
a1 = (6*t0*t1*vxd)/((t0 - t1)*(t0^2 - 2*t0*t1 + t1^2));
a2 = -(3*vxd*(t0 + t1))/((t0 - t1)*(t0^2 - 2*t0*t1 + t1^2));
a3 = (2*vxd)/((t0 - t1)*(t0^2 - 2*t0*t1 + t1^2));

b0 = (vxd*(- t3^3 + 3*t2*t3^2))/((t2 - t3)*(t2^2 - 2*t2*t3 + t3^2));
b1 = -(6*t2*t3*vxd)/((t2 - t3)*(t2^2 - 2*t2*t3 + t3^2));
b2 = (3*vxd*(t2 + t3))/((t2 - t3)*(t2^2 - 2*t2*t3 + t3^2));
b3 = -(2*vxd)/((t2 - t3)*(t2^2 - 2*t2*t3 + t3^2));

Pxdt0 = 0;  % 第1段【原地】结束本体位置
Pxdt1 = Pxdt0 + a0*(t1-t0)+(1/2)*a1*(t1^2-t0^2)+(1/3)*a2*(t1^3-t0^3)+(1/4)*a3*(t1^4-t0^4);  % 第2段【加速】结束本体位置
Pxdt2 = Pxdt1 + vxd*(t2-t1);
Pxdt3 = Pxdt2 + b0*(t3-t2)+(1/2)*b1*(t3^2-t2^2)+(1/3)*b2*(t3^3-t2^3)+(1/4)*b3*(t3^4-t2^4);


%% 分段规划本条前向位置，速度以及加速度

% 原地踏步
if t<t0
    Vxdt = 0;
%     axdt = 0;
    Pxdt = 0;

% 加速阶段
elseif t<t1    
    
    
    Vxdt = a0+a1*t+a2*t^2+a3*t^3;
%     axdt = a1+2*a2*t+3*a3*t^2;
    Pxdt = a0*(t-t0)+(1/2)*a1*(t^2-t0^2)+(1/3)*a2*(t^3-t0^3)+(1/4)*a3*(t^4-t0^4);
    

% 匀速阶段
elseif t<t2
%     vxd = 1;
    Vxdt = vxd;
%     axdt = 0;
    Pxdt = Pxdt1 + Vxdt*(t-t1);
    

% 减速阶段
elseif t<t3    
    Vxdt = b0+b1*t+b2*t^2+b3*t^3;
%     axdt = b1+2*b2*t+3*b3*t^2;
    Pxdt = Pxdt2 + b0*(t-t2)+(1/2)*b1*(t^2-t2^2)+(1/3)*b2*(t^3-t2^3)+(1/4)*b3*(t^4-t2^4);
     
% 原地踏步
elseif t<t4
    Vxdt = 0;
%     axdt = 0;
    Pxdt = Pxdt3;
    
elseif t<t5
    Vxdt = -(a0+a1*(t-t4+t0)+a2*(t-t4+t0)^2+a3*(t-t4+t0)^3);
    Pxdt = Pxdt3 - (a0*(t-t4)+(1/2)*a1*((t-t4+t0)^2-t0^2)+(1/3)*a2*((t-t4+t0)^3-t0^3)+(1/4)*a3*((t-t4+t0)^4-t0^4));

elseif t<t6
    Vxdt = - vxd;
    Pxdt = Pxdt2 + Vxdt*(t-t5);
    
elseif t<t7
    Vxdt = -(b0+b1*(t-t6+t2)+b2*(t-t6+t2)^2+b3*(t-t6+t2)^3);
    Pxdt = Pxdt1 - (b0*(t-t6)+(1/2)*b1*((t-t6+t2)^2-t2^2)+(1/3)*b2*((t-t6+t2)^3-t2^3)+(1/4)*b3*((t-t6+t2)^4-t2^4));
    
else 
    Vxdt = 0;
    Pxdt = 0;   
    
end

TPd = [Pxdt; 0;0;0;0;0];
TVd = [Vxdt; 0;0;0;0;0]; 
Time = t;
end

== matlab function Subsystem/右前腿力//位控制单元 ==
  data: Th2 input double; qd input double; q input double; dot_qd input double; dot_q input double; LegMode input double; Fwd input double; Fwf input double; tau2 output double; Fr output double
function [tau2,Fr]  = SLC(Th2,qd,q,dot_qd,dot_q,LegMode, Fwd,Fwf)

%% 关节角度、足端广义坐标以及雅克比矩阵的计算
th21=Th2(1);
th22=Th2(2);
th23=Th2(3);

% 单腿连杆参数
L1 = 0.35*sqrt(2);
L2 = 0.35*sqrt(2);
R3 = 0.06;

% Jacobian Matrix
J2 = [ -L1*sin(th21 - th22),                   L2*sin(th22) + L1*sin(th21 - th22),                      0;...
          -L1*cos(th21 - th22)*cos(th23), -cos(th23)*(L2*cos(th22) - L1*cos(th21 - th22)), sin(th23)*(L2*sin(th22) + L1*sin(th21 - th22));...
          L1*cos(th21 - th22)*sin(th23),   sin(th23)*(L2*cos(th22) - L1*cos(th21 - th22)),    cos(th23)*(L2*sin(th22) + L1*sin(th21 - th22))];

%% 初始化
 Fr=zeros(3,1);
 Fe = Fwf(4:6);    % 左前腿的足端接触力
 Fd = Fwd(4:6);
 
tau2=zeros(3,1);

%% 单腿力/位控制模式
y = LegMode;
switch(y)
%%%%%%%%%%%%%%%%%%%%%%%%%%%%%
    case 2      % 单腿支撑
        
%        p = diag([2.0  2.0  2.0]);       
%        p = diag([1.5  1.5  1.5]);
%        p = diag([1.4  1.4  1.4]);
%        p = diag([1.3  1.3  1.3]);
%        p = diag([1.2  1.2  1.2]);
       p = diag([1.1  1.1  1.1]);
%        p = diag([1.0  1.0  1.0]);
%        p = diag([0.9  0.9  0.9]);
%        p = diag([0.8  0.8  0.8]);
%        p = diag([0.7  0.7  0.7]);
%        p = diag([0.6  0.6  0.6]);
%        p = diag([0.5  0.5  0.5]);

       F=p*(Fd-Fe);
       Fr=Fd;
       
       tauf=J2'*(F+[0 Fe(2) 0]');
       tau2= -tauf;

%%%%%%%%%%%%%%%%%%%%%%%%%%%%%
    case 1    % 单腿摆动
        kp = diag([7500 7500 7500]);
        kd = diag([120 120 120]);
        
        Fr=zeros(3,1);
        tau2=J2'*(kp*(qd-q)+kd*(dot_qd-dot_q)); 
        
%%%%%%%%%%%%%%%%%%%%%%%%%%%%%
    case 0    % 落后着地
        kp = diag([1000 1500 1000]);
        kd = diag([20 30 20]);
        
        % 在y方向上补偿0.01m
        qd1= qd+[0;-0.01;0];     
        Fr=zeros(3,1);
        tau2=J2'*(kp*(qd1-q)+kd*(dot_qd-dot_q));

%%%%%%%%%%%%%%%%%%%%%%%%%%%%%
     case 3    % 提前着地
      
%        p = diag([1.2  1.2  1.2]);
       p = diag([0.8  0.8  0.8]);
       % y方向零力控制
       Fd=[0;5;0];
       F=p*(Fd-Fe);
       Fr=Fd;
       
       tauf=J2'*(F+[0 Fe(2) 0]');
       tau2=-tauf; 
end

%% 考虑实际情况：输出力矩限幅
Tmax = 500;

if tau2(1)>=Tmax
    tau2(1)=Tmax;
end
if tau2(1)<=-Tmax
    tau2(1)=-Tmax;
end
    
if tau2(2)>=Tmax
    tau2(2)=Tmax;
end
if tau2(2)<=-Tmax
    tau2(2)=-Tmax;
end
    
if tau2(3)>=Tmax
    tau2(3)=Tmax;
end
if tau2(3)<=-Tmax
    tau2(3)=-Tmax;
end

end

== matlab function Subsystem/左后腿力//位控制单元 ==
  data: Th3 input double; qd input double; q input double; dot_qd input double; dot_q input double; LegMode input double; Fwd input double; Fwf input double; tau3 output double; Fr output double
function [tau3,Fr]  = SLC(Th3,qd,q,dot_qd,dot_q,LegMode, Fwd,Fwf)

%% 关节角度、足端广义坐标以及雅克比矩阵的计算
th31=Th3(1);
th32=Th3(2);
th33=Th3(3);

% 单腿连杆参数
L1 = 0.35*sqrt(2);
L2 = 0.35*sqrt(2);
R3 = 0.06;

% Jacobian Matrix
J3 = [ -L1*sin(th31 - th32),                   L2*sin(th32) + L1*sin(th31 - th32),                      0;...
          -L1*cos(th31 - th32)*cos(th33), -cos(th33)*(L2*cos(th32) - L1*cos(th31 - th32)), sin(th33)*(L2*sin(th32) + L1*sin(th31 - th32));...
          -L1*cos(th31 - th32)*sin(th33),  -sin(th33)*(L2*cos(th32) - L1*cos(th31 - th32)),  - cos(th33)*(L2*sin(th32) + L1*sin(th31 - th32))];

%% 初始化
 Fr=zeros(3,1);
 Fe = Fwf(7:9);    % 左前腿的足端接触力
 Fd = Fwd(7:9);
 
tau3=zeros(3,1);

%% 单腿力/位控制模式
y = LegMode;
switch(y)
%%%%%%%%%%%%%%%%%%%%%%%%%%%%%
    case 2      % 单腿支撑
        
%        p = diag([2.0  2.0  2.0]);       
%        p = diag([1.5  1.5  1.5]);
%        p = diag([1.4  1.4  1.4]);
%        p = diag([1.3  1.3  1.3]);
%        p = diag([1.2  1.2  1.2]);
       p = diag([1.1  1.1  1.1]);
%        p = diag([1.0  1.0  1.0]);
%        p = diag([0.9  0.9  0.9]);
%        p = diag([0.8  0.8  0.8]);
%        p = diag([0.7  0.7  0.7]);
%        p = diag([0.6  0.6  0.6]);
%        p = diag([0.5  0.5  0.5]);

       F=p*(Fd-Fe);
       Fr=Fd;
       
       tauf=J3'*(F+[0 Fe(2) 0]');
       tau3= -tauf;

%%%%%%%%%%%%%%%%%%%%%%%%%%%%%
    case 1    % 单腿摆动
        kp = diag([7500 7500 7500]);
        kd = diag([120 120 120]);
        
        Fr=zeros(3,1);
        tau3=J3'*(kp*(qd-q)+kd*(dot_qd-dot_q)); 
        
%%%%%%%%%%%%%%%%%%%%%%%%%%%%%
    case 0    % 落后着地
        kp = diag([1000 1500 1000]);
        kd = diag([20 30 20]);
        
        % 在y方向上补偿0.01m
        qd1= qd+[0;-0.01;0];     
        Fr=zeros(3,1);
        tau3=J3'*(kp*(qd1-q)+kd*(dot_qd-dot_q));

%%%%%%%%%%%%%%%%%%%%%%%%%%%%%
     case 3    % 提前着地
      
%        p = diag([1.2  1.2  1.2]);
       p = diag([0.8  0.8  0.8]);
       % y方向零力控制
       Fd=[0;5;0];
       F=p*(Fd-Fe);
       Fr=Fd;
       
       tauf=J3'*(F+[0 Fe(2) 0]');
       tau3=-tauf; 
end

%% 考虑实际情况：输出力矩限幅
Tmax = 500;

if tau3(1)>=Tmax
    tau3(1)=Tmax;
end
if tau3(1)<=-Tmax
    tau3(1)=-Tmax;
end
    
if tau3(2)>=Tmax
    tau3(2)=Tmax;
end
if tau3(2)<=-Tmax
    tau3(2)=-Tmax;
end
    
if tau3(3)>=Tmax
    tau3(3)=Tmax;
end
if tau3(3)<=-Tmax
    tau3(3)=-Tmax;
end

end

== matlab function Subsystem/右后腿力//位控制单元 ==
  data: Th4 input double; qd input double; q input double; dot_qd input double; dot_q input double; LegMode input double; Fwd input double; Fwf input double; tau4 output double; Fr output double
function [tau4,Fr]  = SLC(Th4,qd,q,dot_qd,dot_q,LegMode, Fwd,Fwf)

%% 关节角度、足端广义坐标以及雅克比矩阵的计算
th41=Th4(1);
th42=Th4(2);
th43=Th4(3);

% 单腿连杆参数
L1 = 0.35*sqrt(2);
L2 = 0.35*sqrt(2);
R3 = 0.06;

% Jacobian Matrix
J4 = [ -L1*sin(th41 - th42),                   L2*sin(th42) + L1*sin(th41 - th42),                      0;...
          -L1*cos(th41 - th42)*cos(th43), -cos(th43)*(L2*cos(th42) - L1*cos(th41 - th42)), sin(th43)*(L2*sin(th42) + L1*sin(th41 - th42));...
          L1*cos(th41 - th42)*sin(th43),   sin(th43)*(L2*cos(th42) - L1*cos(th41 - th42)),    cos(th43)*(L2*sin(th42) + L1*sin(th41 - th42))];

%% 初始化
 Fr=zeros(3,1);
 Fe = Fwf(10:12);    % 左前腿的足端接触力
 Fd = Fwd(10:12);
 
tau4=zeros(3,1);

%% 单腿力/位控制模式
y = LegMode;
switch(y)
%%%%%%%%%%%%%%%%%%%%%%%%%%%%%
    case 2      % 单腿支撑
        
%        p = diag([2.0  2.0  2.0]);       
%        p = diag([1.5  1.5  1.5]);
%        p = diag([1.4  1.4  1.4]);
%        p = diag([1.3  1.3  1.3]);
%        p = diag([1.2  1.2  1.2]);
       p = diag([1.1  1.1  1.1]);
%        p = diag([1.0  1.0  1.0]);
%        p = diag([0.9  0.9  0.9]);
%        p = diag([0.8  0.8  0.8]);
%        p = diag([0.7  0.7  0.7]);
%        p = diag([0.6  0.6  0.6]);
%        p = diag([0.5  0.5  0.5]);

       F=p*(Fd-Fe);
       Fr=Fd;
       
       tauf=J4'*(F+[0 Fe(2) 0]');
       tau4= -tauf;

%%%%%%%%%%%%%%%%%%%%%%%%%%%%%
    case 1    % 单腿摆动
        kp = diag([7500 7500 7500]);
        kd = diag([120 120 120]);
        
        Fr=zeros(3,1);
        tau4=J4'*(kp*(qd-q)+kd*(dot_qd-dot_q)); 
        
%%%%%%%%%%%%%%%%%%%%%%%%%%%%%
    case 0    % 落后着地
        kp = diag([1000 1500 1000]);
        kd = diag([20 30 20]);
        
        % 在y方向上补偿0.01m
        qd1= qd+[0;-0.01;0];     
        Fr=zeros(3,1);
        tau4=J4'*(kp*(qd1-q)+kd*(dot_qd-dot_q));

%%%%%%%%%%%%%%%%%%%%%%%%%%%%%
     case 3    % 提前着地
      
%        p = diag([1.2  1.2  1.2]);
       p = diag([0.8  0.8  0.8]);
       % y方向零力控制
       Fd=[0;5;0];
       F=p*(Fd-Fe);
       Fr=Fd;
       
       tauf=J4'*(F+[0 Fe(2) 0]');
       tau4=-tauf; 
end

%% 考虑实际情况：输出力矩限幅
Tmax = 500;

if tau4(1)>=Tmax
    tau4(1)=Tmax;
end
if tau4(1)<=-Tmax
    tau4(1)=-Tmax;
end
    
if tau4(2)>=Tmax
    tau4(2)=Tmax;
end
if tau4(2)<=-Tmax
    tau4(2)=-Tmax;
end
    
if tau4(3)>=Tmax
    tau4(3)=Tmax;
end
if tau4(3)<=-Tmax
    tau4(3)=-Tmax;
end

end
